simulink model "commhdlQPSKTxRxLoopback_asrun_433fd8da"  (R2025b)
settings: Solver=FixedStepDiscrete  StartTime=0.0  StopTime=stopTime  RelTol=1e-3
PostLoadFcn:
  | hScopeConfig = get_param([gcs '/Receiver/QPSK Rx/Frequency and Time Synchronizer/Symbol Synchronizer/No HDL/QPSK Receiver Eye Diagram'],'ScopeConfiguration');
  | 
  | hScopeConfig.OpenAtSimulationStart = false;
  | hScopeConfig.Visible = false;
  | SamplesPerSymbol = 4;
  | %UpsamplesRx = 1;
  | clear hScopeConfig
InitFcn:
  | commhdlQPSKTxRxModelInit;
  | % Rate bridge: ADRV9002/Jupiter radio runs at 15.36 MHz = 2x the 7.68 MHz
  | % (4 samples/symbol @ Rsym=1.92 MHz) the QPSK Rx requires. The deployed
  | % Receiver must downsample the ADC stream by 2. UpsamplesRx=1 fed the QPSK
  | % Rx 8 sps (2x-upsampled) and broke symbol sync / the loopback bit check.
  | UpsamplesRx = 1;   %% T8 RATE FIX: rail 15.36e6 == ADC bus rate,
  | %% no ingress decimation (was 2 when the rail sat on the 7.68e6 rung)
  | UpsamplesTx = 1;
  | clear simTimingOffset;
StopFcn:
  | if exist('simTimingOffset','var')
  |   disp('Simulation completed');
  |   %QPSKTxRxVerification;
  | end
values from neighbouring files (symbols this model uses):
  Config = commhdlQPSKTxRxParameters    [commhdlQPSKTxRxModelInit.m]
  Rsym = eval(get_param(qpskFindTxInputData(gcs),'Rsym'))    [commhdlQPSKTxRxModelInit.m]
undefined symbols (not defined in the file or in its folder): Add, fsym, randsrc, RandStream, Shift
libraries: hdlsllib x141, simulink x43, dspsigops x34, dsphdlfiltering2 x6, dsphdlsigops2 x4, dsphdlmathfun2 x4, commdigbbndpm3 x4, dspmlti4 x2, commchan3 x1, commrflib2 x1, commcnvcod2 x1
(part 8 of 8)

== matlab function commhdlQPSKTxRxLoopback_asrun_433fd8da/TxRxComposite/Receiver/QPSK Rx/Frequency and Time Synchronizer/Symbol Synchronizer/Loop Filter/LGMux_lt_ss_prop_gain ==
  data: axi input; coeff output; nz output
function [coeff, nz] = lt_ss_prop_gain_mux(axi)
%#codegen
nz = axi ~= uint32(0);
si = bitsliceget(axi, 24, 1);
v  = reinterpretcast(si, numerictype(1, 24, 0));
% clamp IN PLACE (v(:) preserves v's exact type+fimath; assigning v = fi(...)
% rebinds it to a different fimath and breaks Simulink type inference).
if v < -1308048
  v(:) = -1308048;
elseif v > -20438
  v(:) = -20438;
end
coeff = reinterpretcast(v, numerictype(1, 24, 24));
end

== matlab function commhdlQPSKTxRxLoopback_asrun_433fd8da/TxRxComposite/Receiver/QPSK Rx/Frequency and Time Synchronizer/Symbol Synchronizer/Loop Filter/LGMux_lt_ss_integ_gain ==
  data: axi input; coeff output; nz output
function [coeff, nz] = lt_ss_integ_gain_mux(axi)
%#codegen
nz = axi ~= uint32(0);
si = bitsliceget(axi, 24, 1);
v  = reinterpretcast(si, numerictype(1, 24, 0));
% clamp IN PLACE (v(:) preserves v's exact type+fimath; assigning v = fi(...)
% rebinds it to a different fimath and breaks Simulink type inference).
if v < -17440
  v(:) = -17440;
elseif v > -272
  v(:) = -272;
end
coeff = reinterpretcast(v, numerictype(1, 24, 24));
end

== matlab function commhdlQPSKTxRxLoopback_asrun_433fd8da/TxRxComposite/Receiver/QPSK Rx/Automatic Gain Control/Loop Filter/LGMux_lt_agc_loop_gain ==
  data: axi input; coeff output; nz output
function [coeff, nz] = lt_agc_loop_gain_mux(axi)
%#codegen
nz = axi ~= uint32(0);
si = bitsliceget(axi, 32, 1);
v  = reinterpretcast(si, numerictype(0, 32, 0));
% clamp IN PLACE (v(:) preserves v's exact type+fimath; assigning v = fi(...)
% rebinds it to a different fimath and breaks Simulink type inference).
if v < 536871
  v(:) = 536871;
elseif v > 34359738
  v(:) = 34359738;
end
coeff = reinterpretcast(v, numerictype(0, 32, 31));
end

== matlab function commhdlQPSKTxRxLoopback_asrun_433fd8da/TxRxComposite/Receiver/QPSK Rx/Frequency and Time Synchronizer/Coarse Frequency Compensator/CFO step change detector/LGMux_lt_cfo_threshold ==
  data: axi input; firePos output; x input; fireNeg output; nz output
function [firePos, fireNeg, nz] = lt_cfo_threshold_mux(axi, x)
%#codegen
nz = axi ~= uint32(0);
si = bitsliceget(axi, 22, 1);
v  = reinterpretcast(si, numerictype(1, 22, 0));
if v < 3300
  v(:) = 3300;
elseif v > 209712
  v(:) = 209712;
end
thr = reinterpretcast(v, numerictype(1, 22, 21));
firePos = x > thr;
fireNeg = x < (-thr);
end

== matlab function commhdlQPSKTxRxLoopback_asrun_433fd8da/TxRxComposite/Receiver/QPSK Rx/Frequency and Time Synchronizer/Preamble Detector/Correlator/Magnitude Squared and Moving Sum/AccVoter ==
  data: a input; v output; b input; c input
function v = accVoter(a,b,c)
%#codegen
au = reinterpretcast(a, numerictype(0,32,0));
bu = reinterpretcast(b, numerictype(0,32,0));
cu = reinterpretcast(c, numerictype(0,32,0));
vu = bitor(bitand(au,bu), bitor(bitand(au,cu), bitand(bu,cu)));
v = reinterpretcast(vu, numerictype(1,32,28));

== matlab function commhdlQPSKTxRxLoopback_asrun_433fd8da/TxRxComposite/Receiver/QPSK Rx/Frequency and Time Synchronizer/Symbol Synchronizer/Loop Filter Shadow/LGMux_lt_ss_integ_gain ==
  data: axi input; coeff output; nz output
function [coeff, nz] = lt_ss_integ_gain_mux(axi)
%#codegen
nz = axi ~= uint32(0);
si = bitsliceget(axi, 24, 1);
v  = reinterpretcast(si, numerictype(1, 24, 0));
% clamp IN PLACE (v(:) preserves v's exact type+fimath; assigning v = fi(...)
% rebinds it to a different fimath and breaks Simulink type inference).
if v < -17440
  v(:) = -17440;
elseif v > -272
  v(:) = -272;
end
coeff = reinterpretcast(v, numerictype(1, 24, 24));
end

== matlab function commhdlQPSKTxRxLoopback_asrun_433fd8da/TxRxComposite/Receiver/QPSK Rx/Frequency and Time Synchronizer/Symbol Synchronizer/Loop Filter Shadow/LGMux_lt_ss_prop_gain ==
  data: axi input; coeff output; nz output
function [coeff, nz] = lt_ss_prop_gain_mux(axi)
%#codegen
nz = axi ~= uint32(0);
si = bitsliceget(axi, 24, 1);
v  = reinterpretcast(si, numerictype(1, 24, 0));
% clamp IN PLACE (v(:) preserves v's exact type+fimath; assigning v = fi(...)
% rebinds it to a different fimath and breaks Simulink type inference).
if v < -1308048
  v(:) = -1308048;
elseif v > -20438
  v(:) = -20438;
end
coeff = reinterpretcast(v, numerictype(1, 24, 24));
end

== matlab function commhdlQPSKTxRxLoopback_asrun_433fd8da/Transmitter/QPSK Tx/Bit Packetizer/Data Bits FIFO/MATLAB Function1 ==
  data: wr input; full output; rd input; dataBitsPerPacket parameter
function full = fcn(wr,rd,dataBitsPerPacket)
%#codegen
     
    depth = dataBitsPerPacket*2 - 1;
    persistent count;
    if isempty(count)
        count = fi(0,0,nextpow2(depth),0,hdlfimath);
    end

    if wr
        count(:) = count + 1;
    end
    if rd
        count(:) = count - 1;
    end

    full = (count > depth);

end

== matlab function commhdlQPSKTxRxLoopback_asrun_433fd8da/TxRxComposite/Receiver/QPSK Rx/Frequency and Time Synchronizer/Symbol Synchronizer/ShadowScore ==
  data: pP input; pdivCnt output; pS input; iP input; iS input; und input; pdivBeat output; idivBeat output; ipLatch output; isLatch output; strobeFor output; beatCnt output
function [pdivCnt,pdivBeat,idivBeat,ipLatch,isLatch,strobeFor,beatCnt] = shadowScore(pP,pS,iP,iS,und)
%#codegen
persistent pc pb ib ipl isl mg sk gap bt pmPrev
if isempty(pc)
  pc=uint32(0); pb=uint32(0); ib=uint32(0); ipl=uint32(0); isl=uint32(0);
  mg=uint16(0); sk=uint16(0); gap=uint16(0); bt=uint32(0); pmPrev=false;
end
bt = bt + uint32(1);
% P-path upset events (FIR memory self-heals -> every upset = one edge)
pm = (pP ~= pS);
if pm && ~pmPrev
  pc = pc + uint32(1); pb = bt;
end
pmPrev = pm;
% first integrator divergence: latch beat + both raw state words
if ib == uint32(0) && (iP ~= iS)
  ib = bt;
  ipl = uint32(reinterpretcast(iP, numerictype(0,30,0)));
  isl = uint32(reinterpretcast(iS, numerictype(0,30,0)));
end
% symbol-strobe forensic (nominal Underflow spacing 8 beats; >12 = skip)
if gap < uint16(65535), gap = gap + uint16(1); end
if und
  if gap > mg, mg = gap; end
  if gap > uint16(12) && sk < uint16(65535), sk = sk + uint16(1); end
  gap = uint16(0);
end
pdivCnt = pc; pdivBeat = pb; idivBeat = ib; ipLatch = ipl; isLatch = isl;
strobeFor = bitor(bitshift(uint32(mg),16), uint32(sk));
beatCnt = bt;

== matlab function commhdlQPSKTxRxLoopback_asrun_433fd8da/TxRxComposite/Receiver/QPSK Rx/Frequency and Time Synchronizer/Preamble Detector/TaOpsPack ==
  data: taref input; taOps output; udel3 input; psref input; taDiag output
function [taOps, taDiag] = taOpsPack(taref, udel3, psref)
%#codegen
persistent bsm
if isempty(bsm), bsm = uint16(0); end
a = uint32(taref); b = uint32(udel3); p = uint32(psref);
if a == b
  bsm = uint16(0);
elseif bsm < uint16(65535)
  bsm = bsm + uint16(1);
end
taOps  = bitor(bitshift(bitand(a, uint32(16383)), 14), bitand(b, uint32(16383)));
taDiag = bitor(bitshift(uint32(bsm), 16), bitand(p, uint32(16383)));

== matlab function commhdlQPSKTxRxLoopback_asrun_433fd8da/TxRxComposite/Transmitter/Input Data/ByteBitShifter ==
  data: enable input; bit output; reset input; start input; extWord input; extWordAvail input; extWordFirst input; popToggle output
function [bit, popToggle] = byteBitShifterBlk(enable, reset, start, extWord, extWordAvail, extWordFirst)
% Block wrapper around qpskByteBitShifterStrict (the unit-tested single source
% of truth). Persistent state only; the effective enable matches the
% Message Generator chart's active condition (enable && ~reset) so the
% shifter emits bits on exactly the generator's bit steps. pop is
% exported as a toggle (one flip per word latch OR discard) to survive
% the slow->fast rate crossing; upstream edge-detects it into a pulse.
persistent state tog
if isempty(state)
    state = qpskByteBitShifterStrict();
    tog = false;
end
en = logical(enable) && ~logical(reset);
[bit, pop, state] = qpskByteBitShifterStrict(state, en, logical(start), ...
    uint64(extWord), logical(extWordAvail), logical(extWordFirst));
if pop
    tog = ~tog;
end
popToggle = tog;

== matlab function commhdlQPSKTxRxLoopback_asrun_433fd8da/TxRxComposite/Transmitter/Input Data/FEC Tx Encoder K5/TxGateK5 ==
  data: bitIn input; infoBit output; enable input; reset input; start input; encReset output; infoValid output; beatIdx output; frameValid output; frameStart output
function [infoBit, encReset, infoValid, beatIdx, frameValid, frameStart] = fecTxGateK5(bitIn, enable, reset, start)
%#codegen
% sync-semantics (RXROOT E11c): locals in, outputs from locals, persist last.
persistent beat armed;
INFO=uint16(12292); NIN=uint16(12296); PAYLOAD=uint16(24640);
if isempty(beat), beat=uint16(0); armed=false; end
b=beat; a=armed;
infoBit=false; encReset=false; infoValid=false; beatIdx=uint16(0);
frameValid=false; frameStart=false;
en = logical(enable) && ~logical(reset);
if en
  if start, b=uint16(0); a=true; encReset=true; end
  if a
    if b < INFO
      infoBit = logical(bitIn); infoValid = true;
    elseif b < NIN
      infoBit = false;          infoValid = true;   % K-1 zero tail flush
    end
    beatIdx = b; frameValid = true; frameStart = (b==uint16(0));
    if b < PAYLOAD-uint16(1), b=b+uint16(1); else, b=uint16(0); end
  end
end
beat=b; armed=a;

== matlab function commhdlQPSKTxRxLoopback_asrun_433fd8da/TxRxComposite/Transmitter/Input Data/FEC Tx Encoder K5/ConvEncK5 ==
  data: infoBit input; codedPair output; encReset input; infoValid input
function codedPair = fecConvEncK5(infoBit, encReset, infoValid)
%#codegen
persistent sr;
if isempty(sr), sr = false(1,4); end
srUse = sr;
if encReset, srUse = false(1,4); end   % reset-then-advance (zero frame state)
in = logical(infoBit);
s0=in; s1=srUse(1); s2=srUse(2); s3=srUse(3); s4=srUse(4);
g0 = xor(s0, xor(s1, xor(s2, s4)));   % poly 35 oct = 11101
g1 = xor(s0, xor(s3, s4));            % poly 23 oct = 10011
codedPair = [g0; g1];
% state update: advance ONLY on infoValid, else HOLD (anti-zero-stuff gate)
if infoValid
  sr = [in, srUse(1:3)];
else
  sr = srUse;
end

== matlab function commhdlQPSKTxRxLoopback_asrun_433fd8da/TxRxComposite/Transmitter/Input Data/FEC Tx Encoder K5/TxInterleaveK5 ==
  data: codedPair input; dataOut output; infoValid input; beatIdx input; frameValid input; frameStart input
function dataOut = fecTxInterleaveK5(codedPair, infoValid, beatIdx, frameValid, frameStart)
%#codegen
persistent ramA ramB rdBank wptr rrow rcol;
CODED=uint16(24592); COLS=uint16(16); ROWS=uint16(1537);
FILL = logical([1 1 1 1 1 1 1 1 1 0 0 0 0 0 1 1 1 1 0 1 1 1 1 1 0 0 0 1 0 1 1 1 0 0 1 1 0 0 1 0 0 0 0 0 1 0 0 1]);   % 64-bit PN9 filler (T8 fix 6bcaa62)
if isempty(ramA), ramA=fi(zeros(1,24592),0,1,0); ramB=fi(zeros(1,24592),0,1,0); rdBank=false; wptr=uint16(0); rrow=uint16(0); rcol=uint16(0); end
rb=rdBank; w=wptr; rr=rrow; cc=rcol;
dataOut=false;
wr0=uint16(0); wr1=uint16(0); v0=fi(0,0,1,0); v1=fi(0,0,1,0); doW0=false; doW1=false;
if frameValid
  if frameStart, w=uint16(0); rb=~rb; end
  % ---- READ side (previous frame, opposite bank), legacy perm r*COLS+c ----
  % divisionless read address: rr (row 0..ROWS-1) / cc (col 0..COLS-1) are
  % incremental counters, reset on beatIdx==0, advancing +1 row with col carry
  % per in-range beat -- replaces the old per-beat divide-by-ROWS. No divide.
  if beatIdx < CODED
    % precondition: bit-exactness requires a contiguous beatIdx hitting 0 once per
    % frame to re-seed the row/col counters (the old stateless per-beat address
    % arithmetic derived the address from beatIdx alone and needed no such reset).
    if beatIdx == 0, rr = uint16(0); cc = uint16(0); end
    perm = rr*COLS + cc;
    if perm < CODED
      if rb, dataOut = logical(ramB(double(perm)+1)); else, dataOut = logical(ramA(double(perm)+1)); end
    end
    rr = rr + uint16(1);
    if rr == ROWS, rr = uint16(0); cc = cc + uint16(1); end
  else
    dataOut = FILL(double(beatIdx-CODED)+1);   % PN9 filler, beats CODED..2239
  end
  % ---- WRITE side: two coded bits per encoder-advance beat ----
  if infoValid
    if w < CODED, wr0=w; v0=fi(double(codedPair(1)~=0),0,1,0); doW0=true; w=w+uint16(1); end
    if w < CODED, wr1=w; v1=fi(double(codedPair(2)~=0),0,1,0); doW1=true; w=w+uint16(1); end
  end
end
% ---- persist state last (write bank = opposite of read bank) ----
if doW0
  if rb, ramA(double(wr0)+1)=v0; else, ramB(double(wr0)+1)=v0; end
end
if doW1
  if rb, ramA(double(wr1)+1)=v1; else, ramB(double(wr1)+1)=v1; end
end
rdBank=rb; wptr=w; rrow=rr; rcol=cc;

== matlab function commhdlQPSKTxRxLoopback_asrun_433fd8da/TxRxComposite/ByteWordBuffer ==
  data: dataIn input; word output; validIn input; popReq input; firstIn input; avail output; readyNext output; wordFirst output
function [word, avail, readyNext, wordFirst] = byteWordBufferBlk(dataIn, validIn, popReq, firstIn)
% Block wrapper around qpskByteWordBufferSkid (unit-tested single source of
% truth); persistent state only. readyNext = the post-update registered
% ready; an external Delay (IC=1) turns it back into the AXIS tready.
% firstIn/wordFirst carry the in-band first-word marker alongside data.
persistent state
if isempty(state)
    state = qpskByteWordBufferSkid();
end
[word, avail, ~, wordFirst, state] = qpskByteWordBufferSkid(state, uint64(dataIn), ...
    logical(validIn), logical(popReq), logical(firstIn));
readyNext = state.readyReg;

== matlab function commhdlQPSKTxRxLoopback_asrun_433fd8da/Transmitter/QPSK Tx/Bit Packetizer/Data Bits FIFO/RAM Frame Status Indicator ==
  data: push input; out output; pop input; dataBitsPerPacket parameter
function out = fcn(push,pop,dataBitsPerPacket)

   persistent pushCount popCount frameCount;
   if isempty(pushCount)
       pushCount = fi(0,0,nextpow2(dataBitsPerPacket),0,hdlfimath);
       frameCount = fi(0,0,2,0,hdlfimath);
       popCount = fi(0,0,nextpow2(dataBitsPerPacket),0,hdlfimath);
   end
   
   if (pushCount == dataBitsPerPacket-1) && push
       frameCount(:) = frameCount + 1;
   end
   if (popCount == dataBitsPerPacket-1) && pop
       frameCount(:) = frameCount - 1;
   end

   if push
       if pushCount == dataBitsPerPacket - 1
           pushCount(:) = 0;
       else
           pushCount(:) = pushCount + 1;
       end
   end

   if pop 
       if popCount == dataBitsPerPacket - 1
           popCount(:) = 0;
       else
           popCount(:) = popCount + 1;
       end
   end

   out = frameCount;

end

== matlab function commhdlQPSKTxRxLoopback_asrun_433fd8da/TxRxComposite/ByteSerializer ==
  data: bitIn input; word output; bitValid input; start input; ready input; wordTog output; wordLast output; wordFirst output
function [word, wordTog, wordLast, wordFirst] = byteSerializerBlk(bitIn, bitValid, start, ready)
% Block wrapper around qpskByteSerializer (unit-tested single source of
% truth); persistent state only. word/wordLast are HELD stable between
% emissions; wordTog flips once per emitted word so the slow->fast rate
% crossing cannot drop or repeat it -- the 30.72M BeatGate edge-detects
% it into exactly one accepted AXIS beat. Dropped words (ready low at
% completion) do not toggle: drop means NO beat, never a stall.
% K5 kit: 191 words/frame = the first 64*191 of
% the 1084 decoded info bits; the trailing 60 are dropped by start-reset.
persistent state tog heldWord heldLast heldFirst firstNext
if isempty(state)
    state = qpskByteSerializer();
    tog = false; heldWord = uint64(0); heldLast = false;
    heldFirst = true; firstNext = true;
end
% presentation is decoupled from acceptance (ADI S2MM source style):
% the offered beat must refresh on EVERY completed word or the DMA's
% SYNC_TRANSFER_START gate can wait forever on a frozen user flag /
% accept a stale word. ready at the pin only decides acceptance, so
% the core serializer runs with ready=true and unaccepted beats are
% simply superseded.
[w, wv, wl, ~, state] = qpskByteSerializer(state, logical(bitIn), ...
    logical(bitValid), logical(start), true, uint16(191));
if wv
    heldWord = w; heldLast = logical(wl); tog = ~tog;
    heldFirst = firstNext; firstNext = logical(wl);
end
word = heldWord; wordTog = tog; wordLast = heldLast; wordFirst = heldFirst;

== matlab function commhdlQPSKTxRxLoopback_asrun_433fd8da/TxRxComposite/ByteRxFifo ==
  data: word input uint64; outWord output uint64; tog input boolean; wLast input boolean; wFirst input boolean; ready input boolean; valid output boolean; outLast output boolean; outFirst output boolean; ovf output uint32
function [outWord, valid, outLast, outFirst, ovf] = byteRxFifo(word, tog, wLast, wFirst, ready)
%#codegen
% 64-deep elastic FIFO: enqueue on serializer toggle edge, dequeue on
% accepted AXIS beat. Drop-newest + count on full (stall > ~19 ms).
% f1536 SOF-prime guard (TXMUX 2026-07-25): valid is presented only after
% ready has been continuously high for 6 cycles, so the axi_dmac S2MM
% per-descriptor SOF prime (5-cycle latency, replicates a HELD beat x5 =
% the W0x5 dup) never sees a held beat during its prime window.
persistent mem memFl wr rd prev ovfCnt rdyRun
if isempty(wr)
    mem = zeros(64,1,'uint64'); memFl = zeros(64,1,'uint8');
    wr = uint16(0); rd = uint16(0); prev = false; ovfCnt = uint32(0);
    rdyRun = uint8(0);
end
if logical(tog) ~= prev
    nxt = uint16(mod(uint32(wr) + 1, 64));
    if nxt == rd
        rd = uint16(mod(uint32(rd) + 1, 64));
        ovfCnt = ovfCnt + uint32(1);
    end
    mem(uint32(wr)+1)   = uint64(word);
    memFl(uint32(wr)+1) = uint8(wLast) + uint8(2)*uint8(wFirst);
    wr = nxt;
end
prev = logical(tog);
valid = (wr ~= rd) && (rdyRun >= uint8(6));
outWord  = mem(uint32(rd)+1);
fl = memFl(uint32(rd)+1);
outLast  = bitand(fl, uint8(1)) ~= uint8(0);
outFirst = bitand(fl, uint8(2)) ~= uint8(0);
if valid && logical(ready)
    rd = uint16(mod(uint32(rd) + 1, 64));
end
if logical(ready)
    if rdyRun < uint8(255), rdyRun = rdyRun + uint8(1); end
else
    rdyRun = uint8(0);
end
ovf = ovfCnt;

== matlab function commhdlQPSKTxRxLoopback_asrun_433fd8da/TxRxComposite/Receiver/QPSK Rx/Frequency and Time Synchronizer/Preamble Detector/PdTelemetry ==
  data: validIn input boolean; telI output fixdt(1,16,0); dI input int16; dQ input int16; thrEx input boolean; tRef input uint16; tOff input uint16; done input boolean; newPk input boolean; succ input boolean; sync input boolean; armed input boolean; taRef input uint16; accOff input uint16; fifoEnt input uint16; vPop input boolean; tRefLong input uint32; runMax input uint32; heldTs input uint32; telQ output fixdt(1,16,0)
function [telI, telQ] = pdTelemetry(validIn, dI, dQ, thrEx, tRef, tOff, done, newPk, succ, sync, armed, taRef, accOff, fifoEnt, vPop, tRefLong, runMax, heldTs)
%#codegen
persistent slot symCtr beatCnt aDone aNewPk aThrEx aSync aVPop s0 s1 s2 s3 s4 s5 s6
if isempty(slot)
    slot = uint8(7); symCtr = uint32(0); beatCnt = uint8(0);
    aDone = false; aNewPk = false; aThrEx = false; aSync = false; aVPop = false;
    s0 = uint32(0); s1 = uint32(0); s2 = uint32(0); s3 = uint32(0);
    s4 = uint32(0); s5 = uint32(0); s6 = uint32(0);
end
aDone = aDone || done; aNewPk = aNewPk || newPk; aThrEx = aThrEx || thrEx;
aSync = aSync || sync; aVPop = aVPop || vPop;
if beatCnt < uint8(7), beatCnt = beatCnt + uint8(1); end
if validIn
    symCtr = symCtr + uint32(1);
    flags = uint32(aDone) + bitshift(uint32(aNewPk),1) + bitshift(uint32(succ),2) + ...
            bitshift(uint32(aThrEx),3) + bitshift(uint32(aSync),4) + bitshift(uint32(armed),5);
    s0 = bitor(bitor(bitor(bitshift(uint32(14),28), bitshift(uint32(bitand(tRef,uint16(2047))),17)), ...
         bitshift(uint32(bitand(tOff,uint16(2047))),6)), flags);
    s1 = bitor(bitshift(uint32(reinterpretcast(dI,numerictype(0,16,0))),16), ...
         uint32(reinterpretcast(dQ,numerictype(0,16,0))));
    s2 = bitor(bitor(bitor(bitshift(uint32(bitand(taRef,uint16(2047))),21), ...
         bitshift(uint32(bitand(accOff,uint16(2047))),10)), ...
         bitshift(uint32(bitand(fifoEnt,uint16(511))),1)), uint32(aVPop));
    s3 = tRefLong;
    s4 = runMax;
    s5 = heldTs;
    s6 = bitor(bitor(bitshift(uint32(165),24), bitshift(uint32(bitand(uint16(beatCnt),uint16(7))),21)), ...
         bitand(symCtr,uint32(2097151)));
    aDone = false; aNewPk = false; aThrEx = false; aSync = false; aVPop = false;
    beatCnt = uint8(0);
    slot = uint8(0);
end
switch slot
  case uint8(0), w = s0;
  case uint8(1), w = s1;
  case uint8(2), w = s2;
  case uint8(3), w = s3;
  case uint8(4), w = s4;
  case uint8(5), w = s5;
  case uint8(6), w = s6;
  otherwise,     w = uint32(0);
end
if slot < uint8(7), slot = slot + uint8(1); end
telI = reinterpretcast(uint16(bitshift(w, -16)), numerictype(1,16,0));
telQ = reinterpretcast(uint16(bitand(w, uint32(65535))), numerictype(1,16,0));

== matlab function commhdlQPSKTxRxLoopback_asrun_433fd8da/Receiver/QPSK Rx/Frequency and Time Synchronizer/Packet Controller/sample discard controller ==
  data: dataIn input; validIn input; dataOut output; startIn input; endIn input; startOut output; endOut output; validOut output
function [dataOut,startOut,endOut,validOut] = controller(dataIn,validIn,startIn,endIn)
%#codegen

   persistent active dataOutReg validOutReg startOutReg endOutReg;
   if isempty(active)
      active  = false;
      dataOutReg = cast(0,'like',dataIn);
      validOutReg = false;
      startOutReg = false;
      endOutReg = false;
   end
   
   dataOut = dataOutReg;
   validOut = validOutReg;
   startOut = startOutReg;
   endOut = endOutReg;
   
   startOutReg = startIn;
   endOutReg = endIn;
   
   if startIn
       active = true;
   end
   
   if active
       dataOutReg(:) = dataIn;
       validOutReg = validIn;
   else
       dataOutReg(:) = 0;
       validOutReg = false;
   end
   
   if endIn
       if active 
           endOutReg = true;
       else
           endOutReg = false;
       end
       active = false;
   end
end

== matlab function commhdlQPSKTxRxLoopback_asrun_433fd8da/Receiver/QPSK Rx/Frequency and Time Synchronizer/Symbol Synchronizer/Interpolation Control ==
  data: mu output; Delta input; Underflow output
function [mu,Underflow] = Interpolation_ctrl(Delta)
% Implementation of modulo-1 counter for interpolation control listed in
% Figure 8.4.19 of "Digital Communications - A Discrete-Time Approach"
% by Michael Rice. See design details in Chapter 8.4.3 of the same book.
% 
% Input:
%   Delta - Loop filter output. If loop is in lock, delta would be small
% Output:
%   Underflow - Indicator of counter underflow. This is the strobe signal
%               for downstream processing
%   mu - Difference between actual sampling instant and the optimal instant,
%        between zero and one
%#codegen

% countReg - Counter value delayed by 1 sample
% muReg - The estimated timing error normalized by half QPSK symbols

   mask = fi(1-2^(-10),1,11,10);
   
   persistent countReg underflowReg muReg;
   if isempty(countReg)
       countReg  = fi(0,1,11,10);
       muReg = fi(0,1,11,10);
       underflowReg = false;
   end
   
   
   Underflow = underflowReg;
   mu = muReg;   
   
   
      % T8.4 anti-wedge clamp: if Delta <= -0.125 the decrementing counter
   % never underflows (strobes stop FOREVER -- Class-4 wedge / Class-1
   % episode mechanism; see tb_timing_wedge.v). Bound Delta so the
   % counter always decrements by >= 1 LSB.
   wlim = fi(255/1024,1,11,10);
   if Delta > wlim
       Delta = wlim;
   elseif Delta < -wlim
       Delta = fi(-255/1024,1,11,10);
   end
   counter = bitand(mask,countReg)-Delta-fi(0.25,1,11,10); % decrementing counter
   
   % if countReg is a nonnegative number,
   % then mod(countReg,1) equals the fractional part of countReg
   if counter < 0
       underflowReg = true;
       muReg = bitshift(bitand(mask,countReg),2);
       countReg = fi(counter+1,1,11,10);% create underflow to counter
   else
       underflowReg = false;
       countReg = fi(counter,1,11,10);
   end
   


end

== matlab function commhdlQPSKTxRxLoopback_asrun_433fd8da/Receiver/QPSK Rx/Frequency and Time Synchronizer/Preamble Detector/Correlator/ThresholdLimiter ==
  settings: fimath=hdlfimath
  data: x input; y output
function y = applyLowerLimit(x)
    % Apply a lower limit to the threshold.
    %#codegen
    
    % Threshold is computed by summing across 63 samples.
    % Set lower limit to be equivalent of all 63 samples
    % having their LSB set to 1 and all others set to 0. 
    lowerLimit = cast(0.01, 'like', x);
    
    if x < lowerLimit
        y = lowerLimit;
    else
        y = x;
    end
end

== matlab function commhdlQPSKTxRxLoopback_asrun_433fd8da/Transmitter/Input Data/Message Generator/MATLAB Function ==
  data: enable input; reset input; out output; start output; stop output; valid output; count_out output; msg_count_out output
function [out, start, stop, valid, count_out, msg_count_out] = msggen(enable, reset)

persistent indexCount;
persistent toggle;
persistent msgCount;
persistent msgCountAll;
persistent msgCountBitIndex;

if isempty(indexCount) || isempty(toggle) || isempty(msgCount) || isempty(msgCountBitIndex) || isempty(msgCountAll)
    indexCount = uint32(0);
    msgCount = uint32(1);
    msgCountAll = uint32(1);
    msgCountBitIndex = uint8(0);
    toggle = false;
end

%% Constants
strAscii = dec2bin('ADI Hello World', 8);
msgarray = reshape(strAscii', [1, numel(strAscii)]);
msgbits = logical(msgarray - 48);
msgbitsLen = length(msgbits);

fullMessageLen = uint32(2240-1); % Need the -1 to eat the feedback delay

% Bit counter
% N = 8;% 8-bit counter
% mask = uint32(2^N - 1);
% for k = 1:300
%     msgCount = bitand(msgCount + uint32(1), mask);   % wraps 255 -> 0
% end

%% Logic
if enable && ~reset
    % Set out data
    if indexCount < msgbitsLen % Insert msg
        out = msgbits(indexCount + 1);
        msgCountBitIndex = uint8(0);
    else % Zero padding: varying filler (counter digit + toggle bits)
        % caused periodic false-lock error bursts in the deployed BIST;
        % zero-padded payload matches the verified host golden structure.
        out = false;
        msgCountBitIndex = uint8(0);
    end

    % Flags
    start = indexCount == uint32(0);
    stop = indexCount == fullMessageLen;
    valid = true;

    % Counters
    if fullMessageLen == indexCount
        if msgCount >= 9
            msgCount = uint32(1);
        else
            msgCount = msgCount +  1;
            msgCountAll = msgCountAll + 1;
        end
    end
    if indexCount <= fullMessageLen
        indexCount = indexCount + 1;
    end

else % Enable == false

    if reset
        indexCount = uint32(0);
        % msgCount = uint32(0);
        msgCountBitIndex = uint8(0);
        toggle = false;
    end
    out = false;
    start = false;
    stop = false;
    valid = false;
end

if isempty(indexCount)
    count_out = uint32(0);
else
    count_out = indexCount;
end

msg_count_out = msgCountAll;
